simulink model "project2"  (R2017b)
settings: Solver=VariableStepDiscrete  StartTime=0.0  StopTime=10.0  RelTol=1e-3
undefined symbols (not defined in the file): Ion, Lithium
libraries: powerlib x6, electricdrivelib x1, re_lib x1, powerlib_meascontrol x1
settings Model: Creator=RICHARD MARTIN  LastModifiedBy=RICHARD MARTIN

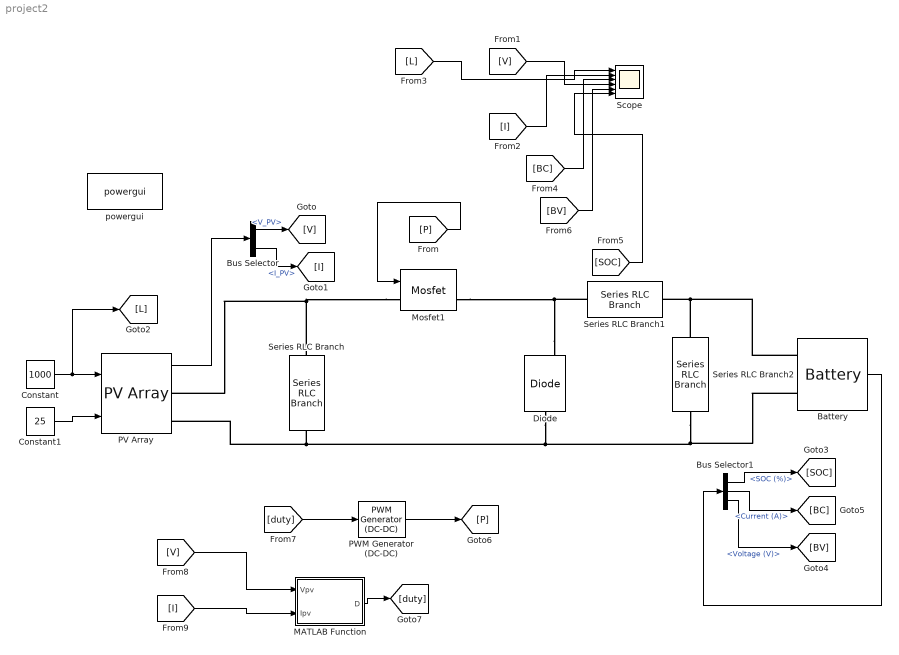
== system project2 ==
  Battery : electricdrivelib/Extra Sources/Battery  BatType=Lithium-Ion  ShowTempParam=off  ThermalPreset=no  ShowAgeParam=off  NomV=7.2  NomQ=5.4  SOC=100  Batt_Tr=30  PresetModel=off  MaxQ=5.4  MinV=5.4  FullV=8.3807  Dis_rate=2.3478  R=0.013333  Normal_OP=4.8835  expZone="[7.7788      0.2653]"  current=[6.5 13 32.5]  Units=Time  Tci=20  NomT=20  T2=-30  MaxQ2=4.8  FullV2=7.1  Normal_OP2=5.655  expZone2="[6.58           1]"  Rca=0.6  ti=2000  Dp=0  Neq0=0  Tsim=1e6  Ta1=25  Qeol=5.4*0.9  Reol=0.013333*1.2  Char_age=[2.3478, 3]  Dis_age=[2.3478, 10]  N1=1500  N2=10500  N3=1000  N4=1400  Ta2=45  N5=950
  Bus Selector : BusSelector  OutputSignals=V_PV,I_PV
  Bus Selector1 : BusSelector  OutputSignals=SOC (%),Current (A),Voltage (V)
  Constant : Constant  Value=1000
  Constant1 : Constant  Value=25
  Diode : powerlib/Power Electronics/Diode  Ron=0.001  Lon=0  Vf=0.8  IC=0  UseSnubber=0  Rs=500  Cs=250e-9  Measurements=on
  MATLAB Function : MATLAB Function  TreatAsAtomicUnit=on
  Mosfet1 : powerlib/Power Electronics/Mosfet  Ron=0.1  Lon=0  Rd=0.01  Vfd=0  IC=0  Rs=1e5  Cs=inf  Measurements=on
  PV Array : re_lib/Solar/PV Array  Npar=5  Nser=1  PlotType=array @ 1000 W/m2 & specified temperatures  S_vec="[ 1000  500  100 ]"  Temp_C_vec="[ 45 25  ]"  ModuleName=1Soltech 1STH-215-P  PlotWhenSelected=off  Pm=213.15  Ncell=60  Voc=36.3  Isc=7.84  Vm=29  Im=7.35  beta_Voc_pc=-0.36099  alpha_Isc_pc=0.102  beta_Voc=-0.13104  alpha_Isc=0.007997  IL=7.8649  I0=2.9259e-10  nI=0.98117  Rsh=313.3991  Rs=0.39383  BAL=on  Tc=1e-6  Tfilter=5e-5
  PWM Generator (DC-DC) : powerlib_meascontrol/Pulse & Signal Generators/PWM Generator (DC-DC)  Fsw=5000  Ts=10e-6
  Scope : Scope  NumInputPorts=6
  Series RLC Branch : powerlib/Elements/Series RLC Branch  LConnTagsString=__new0  RConnTagsString=__new0  BranchType=RC  Resistance=0.0001  Inductance=0  SetiL0=off  InitialCurrent=0  Capacitance=1000e-6  Setx0=off  InitialVoltage=0  Measurements=None
  Series RLC Branch1 : powerlib/Elements/Series RLC Branch  LConnTagsString=__new0  RConnTagsString=__new0  BranchType=L  Resistance=0.0001  Inductance=0.783e-3  SetiL0=off  InitialCurrent=0  Capacitance=1000e-6  Setx0=off  InitialVoltage=0  Measurements=None
  Series RLC Branch2 : powerlib/Elements/Series RLC Branch  LConnTagsString=__new0  RConnTagsString=__new0  BranchType=C  Resistance=0.0001  Inductance=0.783e-6  SetiL0=off  InitialCurrent=0  Capacitance=364e-6  Setx0=off  InitialVoltage=0  Measurements=None
  powergui : powerlib/powergui  Priority=1  SimulationMode=Discrete  SampleTime=1e-05  frequency=60  Iterations=50  frequencyindice=0  Pbase=100e6  ErrMax=1e-4  UnitsV=kV  UnitsW=MW  buscounter=0  FunctionMessages=off  echomessages=off  EnableUseOfTLC=off  CurrentSourceSwitches=off  DisableSnubberDevices=off  DisableRonSwitches=off  DisableVfSwitches=off  DisplayEquations=off  SolverType=Tustin/Backward Euler (TBE)  Interpol=off  ExternalGateDelay=off  methode=off  Ts=100  x0status=blocks  SPID=on  SwTol=0  HookPort=off  RestoreLinks=warning  ResistiveCurrentMeasurement=off  Frange=[0:2:500]  Ylog=off  Xlog=on  ShowGrid=off  save=off  variable=ZData  structure=0  ZoomFFT=off  StartTime=0.0  cycles=1  DisplayStyle=1  fundamental=60  FreqAxis=off  MaxFrequency=1000  frequencyindicesteady=1  RmsSteady=1  display=off
  wires:
  PV Array/1 -> Bus Selector/1
  Bus Selector/1 -> [V]  "<V_PV>"
  Bus Selector/2 -> [I]  "<I_PV>"
  Constant/1 -> [L], PV Array/1
  Constant1/1 -> PV Array/2
  [P] -> Mosfet1/1
  Battery/1 -> Bus Selector1/1
  Bus Selector1/1 -> [SOC]  "<SOC (%)>"
  Bus Selector1/2 -> [BC]  "<Current (A)>"
  Bus Selector1/3 -> [BV]  "<Voltage (V)>"
  [V] -> Scope/4
  [I] -> Scope/2
  [BC] -> Scope/3
  [BV] -> Scope/5
  [SOC] -> Scope/6
  [L] -> Scope/1
  PWM Generator (DC-DC)/1 -> [P]
  [duty] -> PWM Generator (DC-DC)/1
  MATLAB Function/1(D) -> [duty]
  [V] -> MATLAB Function/1(Vpv)
  [I] -> MATLAB Function/2(Ipv)
  connections:
  Diode/LConn1 -- PV Array/RConn2 -- Series RLC Branch/RConn1 -- Battery/LConn2 -- Series RLC Branch2/RConn1
  Mosfet1/LConn1 -- PV Array/RConn1 -- Series RLC Branch/LConn1
  Diode/RConn1 -- Mosfet1/RConn1 -- Series RLC Branch1/RConn1
  Series RLC Branch1/LConn1 -- Series RLC Branch2/LConn1 -- Battery/LConn1

== matlab function project2/MATLAB Function ==
  data: Vpv input; D output; Ipv input
function D = Pand0(Vpv,Ipv)

persistent Dprev Pprev Vprev
if isempty(Dprev)
    Dprev = 0.7;
    Vprev = 190;
    Pprev = 2000;
end
deltaD = 125e-6;

Ppv = Vpv * Ipv;

if(Ppv-Pprev) ~=0
  if(Ppv - Pprev) >0
    if(Vpv - Vprev)>0
        D=Dprev - deltaD;
    else
        D=Dprev + deltaD;
    end
  else
    if (Vpv-Vprev)>0
        D= Dprev+deltaD; 
    else
        D=Dprev - deltaD;
    end
  end
else
    D=Dprev;
end

Dprev = D;
Vprev= Vpv;
Pprev =Ppv;
